simulink model "UnitTest"  (R2022b)
settings: Solver=VariableStepAuto  StartTime=0.0  StopTime=10  RelTol=1e-3
values from neighbouring files (symbols this model uses):
  b = 15    [Init_Celc.m]
  cmaxfit = -4.70546620480099*(10.^-8)*temp.^4+	3.49662102291610*(10.^-6)*temp.^3 +	0.00209286380926111*temp.^2	-0.0176104377910828*temp+	0.0300191236909972    [Init_Celc.m]
  f = 0.001    [Init_Celc.m]
  J = 0.0015    [Init_Celc.m]
  r = 0.75    [Init_Celc.m]
  rho = 1.20    (= 1.2)    [Init_Celc.m]
  s = pi*r.^2    [Init_Celc.m]
  temp = (1:vit_syn/40:vit_syn)    [Init_Celc.m]
settings Model: Creator=ZinouAb  LastModifiedBy=ZinouAb

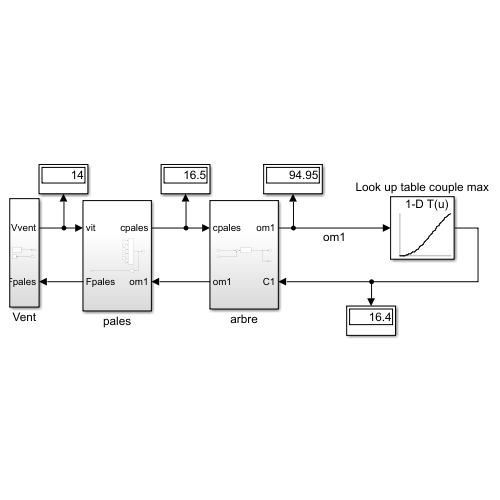
[thumbnail: Simulink's stored preview of the top-level diagram]
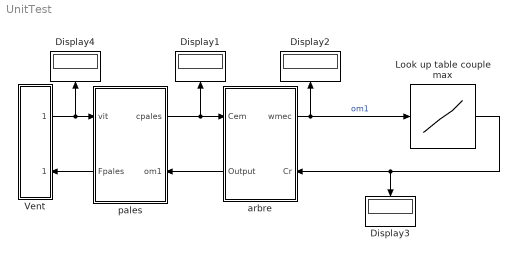
== system UnitTest ==
  Display{1..4} (4 alike) : Display
  Look up table couple max : Lookup_n-D  NumberOfTableDimensions=1  BreakpointsForDimension1=temp  Table=cmaxfit  InternalRulePriority=Speed  RndMeth=Simplest
  Vent : Subsystem
      settings: PortSchema="{\"entries\":[{\"content\":{\"sides\":[{\"content\":{\"connectorIds\":[]},\"type\":\"ConnectorPlacement.EquallySpacedRectSide\",\"uuid\":\"be9e5db0-62db-41cd-9655-d6d790779573\"},{\"content\":{\"connectorIds\":[\"Out1\",\"In1\"],\"side\":\"RIGHT\"},\"type\":\"ConnectorPlacement.EquallySpacedRectSide\",\"uuid\":\"b5e788b3-1e5f-4899-a162-7a564b67bc63\"},{\"content\":{\"connectorIds\":[],\"side\":\"TOP\"},\"type\":\"ConnectorPlacement.EquallySpacedRectSide\",\"uuid\":\"cac5ef03-1794-4810-a86f-81d9785b0908\"}]},\"type\":\"ConnectorPlacement.EquallySpacedConnector\",\"uuid\":\"fdefeacd-144d-477b-b7c5-141053c244e1\"}],\"packageUris\":[\"http://schema.mathworks.com/mf0/Connector/R2020b\"],\"version\":\"1.0\"}"
  arbre : Subsystem
      settings: PortSchema="{\"entries\":[{\"content\":{\"sides\":[{\"content\":{\"connectorIds\":[\"In1\",\"Out2\"]},\"type\":\"ConnectorPlacement.EquallySpacedRectSide\",\"uuid\":\"b8908f99-787f-4ebd-a8c4-361ef654133e\"},{\"content\":{\"connectorIds\":[\"Out1\",\"In2\"],\"side\":\"RIGHT\"},\"type\":\"ConnectorPlacement.EquallySpacedRectSide\",\"uuid\":\"e7049b46-0747-4182-8580-458ffa90f1c3\"},{\"content\":{\"connectorIds\":[],\"side\":\"TOP\"},\"type\":\"ConnectorPlacement.EquallySpacedRectSide\",\"uuid\":\"013bc89f-8670-489b-af07-681a8894793a\"}]},\"type\":\"ConnectorPlacement.EquallySpacedConnector\",\"uuid\":\"dba8a148-0e4d-4308-b676-65e370746724\"}],\"packageUris\":[\"http://schema.mathworks.com/mf0/Connector/R2020b\"],\"version\":\"1.0\"}"
  pales : Subsystem
      settings: PortSchema="{\"entries\":[{\"content\":{\"sides\":[{\"content\":{\"connectorIds\":[\"In1\",\"Out2\"]},\"type\":\"ConnectorPlacement.EquallySpacedRectSide\",\"uuid\":\"2ecec5eb-5bb6-4f05-bbbb-1a51ae98f814\"},{\"content\":{\"connectorIds\":[\"Out1\",\"In2\"],\"side\":\"RIGHT\"},\"type\":\"ConnectorPlacement.EquallySpacedRectSide\",\"uuid\":\"ddc3d36f-31b1-43d5-b617-6997f76d08f1\"},{\"content\":{\"connectorIds\":[],\"side\":\"TOP\"},\"type\":\"ConnectorPlacement.EquallySpacedRectSide\",\"uuid\":\"42603242-cda1-4bb2-8cac-1b3409f39577\"}]},\"type\":\"ConnectorPlacement.EquallySpacedConnector\",\"uuid\":\"febb8687-16a8-4638-bd43-9ebf443fd4bd\"}],\"packageUris\":[\"http://schema.mathworks.com/mf0/Connector/R2020b\"],\"version\":\"1.0\"}"
  wires:
  Vent/1(Out1) -> Display4/1, pales/1(vit)
  arbre/1(wmec) -> Display2/1, Look up table couple max/1  "om1"
  pales/1(cpales) -> arbre/1(Cem), Display1/1
  Look up table couple max/1 -> Display3/1, arbre/2(Cr)
  pales/2(Fpales) -> Vent/1(In1)
  arbre/2(Output) -> pales/2(om1)

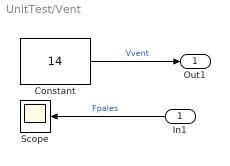
== system UnitTest/Vent ==
  In1 : Inport
  Constant : Constant  Value=14
  Scope : Scope
  Out1 : Outport
  wires:
  In1/1 -> Scope/1  "Fpales"
  Constant/1 -> Out1/1  "Vvent"

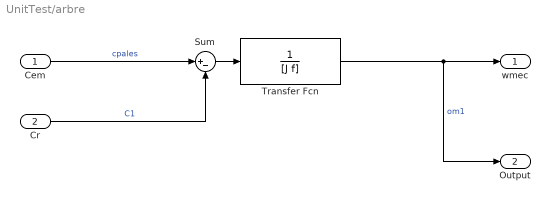
== system UnitTest/arbre ==
  Cem : Inport
  Cr : Inport  Port=2
  Sum : Sum  Inputs=|+-
  Transfer Fcn : TransferFcn  Denominator=[J f]
  wmec : Outport
  Output : Outport  Port=2
  wires:
  Cem/1 -> Sum/1  "cpales"
  Sum/1 -> Transfer Fcn/1
  Cr/1 -> Sum/2  "C1"
  Transfer Fcn/1 -> Output/1, wmec/1  "om1"

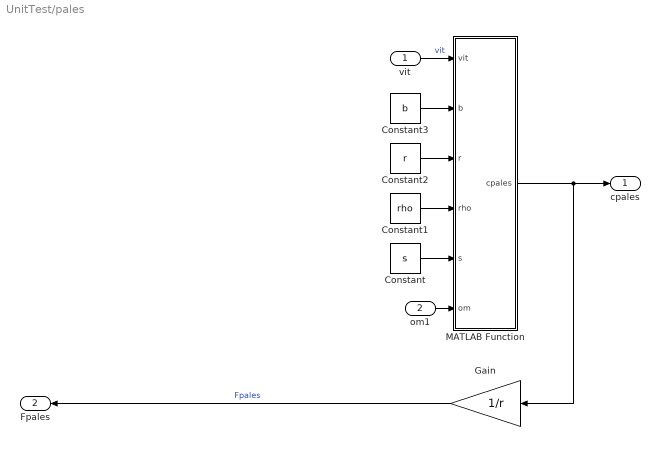
== system UnitTest/pales ==
  vit : Inport
  om1 : Inport  Port=2
  Constant : Constant  Value=s
  Constant1 : Constant  Value=rho
  Constant2 : Constant  Value=r
  Constant3 : Constant  Value=b
  Gain : Gain  Gain=1/r
  MATLAB Function : MATLAB Function  TreatAsAtomicUnit=on
  cpales : Outport
  Fpales : Outport  Port=2
  wires:
  vit/1 -> MATLAB Function/1(vit)  "vit"
  om1/1 -> MATLAB Function/6(om)
  Constant2/1 -> MATLAB Function/3(r)
  MATLAB Function/1(cpales) -> Gain/1, cpales/1
  Gain/1 -> Fpales/1  "Fpales"
  Constant/1 -> MATLAB Function/5(s)
  Constant1/1 -> MATLAB Function/4(rho)
  Constant3/1 -> MATLAB Function/2(b)

== matlab function UnitTest/pales/MATLAB Function ==
  data: vit input; b input; cpales output; r input; rho input; s input; om input
function cpales = fcn(vit,b,r,rho,s,om)

    lamb=r*om/vit;
  
    if lamb==0    % Pour éviter d'avoir une division par zero par la suite
        lamb=0.001;
    end
        lamb1=1/((1/(lamb+0.089*b))-(0.035/(b^3+1)));
        Cp=0.5*(116/lamb1-0.4*(b-5))*exp(-16.5/lamb1);
        Ct=Cp/lamb;
        cpales=0.5*rho*Ct*r*s*vit^2;





end
